simulink model "controller13_AIS"  (R2020b)
settings: Solver=FixedStepDiscrete  StartTime=0.0  StopTime=inf  RelTol=1e-3
values from neighbouring files (symbols this model uses):
  ctr = make_controller()    [setup_controller_with_functions.m]
  mdl = make_model(flight_time)    [setup_controller_with_functions.m]
  ukf_P0_flat = UKF.flatten_matrix(ukf_sys.P0)    [controller_setup_ukf.m]
  ukf_prediction_time = 0.015    [controller_setup_ukf.m]
  ukf_s0 = ukf_sys.s0    [controller_setup_ukf.m]
  ukf_sys = UKF.initialize_ukf_sys(rbt, mdl, ukf_params)    [controller_setup_ukf.m]
  ukf_use_prediction = 1    [controller_setup_ukf.m]
undefined symbols (not defined in the file or in its folder): ctr1, ctr2, DiscIntNeverNeededParam, flt, IO397, rbt1, rbt2, rsim1, rsim2, som, traj2
libraries: simulink x63, slrealtimeloglib x21, slrealtimetgmanagement x8, slrealtimeseriallib x5, speedgoatlib_fpga_analog_io x4, slrealtimeutilitieslib x3, dspfdesign x2, speedgoatlib_fpga x2, slrealtimeiplib x2, speedgoatlib_fpga_dio x1
(part 4 of 5)

== system controller13_AIS/Measurement manager 2/safety check system/landing condition ==
  z : Inport
  Add : Sum  Inputs=+--
  SaturatingRamp1 : DiscreteIntegrator  gainval=1  SampleTime=-1  UpperSaturationLimit=1  LowerSaturationLimit=0  ICPrevOutput=DiscIntNeverNeededParam  ICPrevScaledInput=DiscIntNeverNeededParam
  constant : Constant
  constant1 : Constant  Value=2
  constant2 : Constant  Value=mdl.i_delay
  landing_cond : MATLAB Function  TreatAsAtomicUnit=on  SystemSampleTime=mdl.T
  en : Outport
  wires:
  SaturatingRamp1/1 -> Add/1
  constant/1 -> SaturatingRamp1/1
  constant1/1 -> Add/2
  constant2/1 -> Add/3
  Add/1 -> landing_cond/2(time_cond)
  z/1 -> landing_cond/1(alt)
  landing_cond/1(en) -> en/1

== system controller13_AIS/signal generator 1/Bias_Signal/AveragedBias ==
  note: To avoid having signal "jump",
      | we want SMOOTH transitions
      | in frequency (i.e., a weighted sum
      | of current freq and freq some delta t ago)
  note: time constant = 0.002sec
  In1 : Inport
  Discrete Transfer Fcn : DiscreteTransferFcn  Numerator=[0.05]  Denominator=[1 -.95]
  Out1 : Outport
  wires:
  In1/1 -> Discrete Transfer Fcn/1
  Discrete Transfer Fcn/1 -> Out1/1

== system controller13_AIS/signal generator 1/Bias_Signal/SIgnalForRamp_binary ==
  note: Should output 1 or -1,
      | so signal ramps UP to 1
      | or DOWN to 0.
  In1 : Inport
  Add : Sum  Inputs=+-
  Compare To Zero : simulink/Logic and Bit Operations/Compare To Zero  relop=>  OutDataTypeStr=uint8  ZeroCross=off
  Constant : Constant
  Data Type Conversion : DataTypeConversion  OutDataTypeStr=double
  Gain : Gain  Gain=2
  Out1 : Outport
  wires:
  In1/1 -> Compare To Zero/1
  Compare To Zero/1 -> Data Type Conversion/1
  Gain/1 -> Add/1
  Constant/1 -> Add/2
  Add/1 -> Out1/1
  Data Type Conversion/1 -> Gain/1

== system controller13_AIS/signal generator 1/Drive_Signal1/AveragedAmp_filtered ==
  note: To avoid having signal "jump",
      | we want SMOOTH transitions
      | in frequency (i.e., a weighted sum
      | of current freq and freq some delta t ago)
  note: time constant 0.002sec
      | for 10kHz samping
  In1 : Inport
  Discrete Transfer Fcn : DiscreteTransferFcn  Numerator=[0.05]  Denominator=[1 -.95]
  Out1 : Outport
  wires:
  In1/1 -> Discrete Transfer Fcn/1
  Discrete Transfer Fcn/1 -> Out1/1

== system controller13_AIS/signal generator 1/Drive_Signal1/AveragedOffset_filtered ==
  note: To avoid having signal "jump",
      | we want SMOOTH transitions
      | in frequency (i.e., a weighted sum
      | of current freq and freq some delta t ago)
  note: c
  note: time constant 0.02sec
      | for 10kHz samping
  In1 : Inport
  Discrete Transfer Fcn : DiscreteTransferFcn  Numerator=[0.05]  Denominator=[1 -.95]
  Out1 : Outport
  wires:
  In1/1 -> Discrete Transfer Fcn/1
  Discrete Transfer Fcn/1 -> Out1/1

== system controller13_AIS/signal generator 1/Drive_Signal1/AveragedTau_filtered ==
  note: To avoid having signal "jump",
      | we want SMOOTH transitions
      | in frequency (i.e., a weighted sum
      | of current freq and freq some delta t ago)
  note: time constant 0.002sec
      | for 10kHz samping
  In1 : Inport
  Discrete Transfer Fcn : DiscreteTransferFcn  Numerator=[0.05]  Denominator=[1, -0.95]
  Out1 : Outport
  wires:
  In1/1 -> Discrete Transfer Fcn/1
  Discrete Transfer Fcn/1 -> Out1/1

== system controller13_AIS/signal generator 1/Drive_Signal1/SignalForRamp_binary ==
  note: Should output 1 or -1,
      | so signal ramps UP to 1
      | or DOWN to 0.
  In1 : Inport
  Add : Sum  Inputs=+-
  Compare To Zero : simulink/Logic and Bit Operations/Compare To Zero  relop=>  OutDataTypeStr=uint8  ZeroCross=off
  Constant : Constant
  Data Type Conversion : DataTypeConversion  OutDataTypeStr=double
  Gain : Gain  Gain=2
  Out1 : Outport
  wires:
  In1/1 -> Compare To Zero/1
  Compare To Zero/1 -> Data Type Conversion/1
  Gain/1 -> Add/1
  Constant/1 -> Add/2
  Add/1 -> Out1/1
  Data Type Conversion/1 -> Gain/1

== system controller13_AIS/signal generator 1/Drive_Signal1/SignalForSin_binary ==
  note: We want this to stay "high" for 1
      | second after the actual "enable"
      | is turned off...
  In1 : Inport
  Compare To Zero : simulink/Logic and Bit Operations/Compare To Zero  relop=>  OutDataTypeStr=uint8  ZeroCross=off
  Data Type Conversion : DataTypeConversion  OutDataTypeStr=double
  Out1 : Outport
  wires:
  In1/1 -> Compare To Zero/1
  Compare To Zero/1 -> Data Type Conversion/1
  Data Type Conversion/1 -> Out1/1

== system controller13_AIS/signal generator 1/Drive_Signal1/Subsystem ==
  note: positive value pushes the left wing forward
  split cycle mu : Inport
  In2 : Inport  Port=2
  1-mu : Sum  Inputs=+-
  2f : Gain  Gain=2
  2nd harmonic : Trigonometry  OutputSignalType=real
  2pi : Gain  Gain=2*pi
  Abs1 : Abs
  Add : Sum
  Constant : Constant
  combined sines : Sum
  deg to rad : Gain  Gain=pi/180
  f : Gain  Gain=-1
  first harmonic : Trigonometry  OutputSignalType=real
  omega*t : DiscreteIntegrator  SampleTime=-1  ICPrevOutput=DiscIntNeverNeededParam  ICPrevScaledInput=DiscIntNeverNeededParam
  phase offset : Constant  Value=0
  signal with gain1 : Product  RndMeth=Zero
  signal with gain2 : Product  RndMeth=Zero
  split cycle signal : Outport
  wires:
  2f/1 -> 2nd harmonic/1
  first harmonic/1 -> signal with gain1/2
  Constant/1 -> 1-mu/1
  split cycle mu/1 -> f/1, Abs1/1
  1-mu/1 -> signal with gain1/1
  2nd harmonic/1 -> signal with gain2/2
  signal with gain1/1 -> combined sines/1
  signal with gain2/1 -> combined sines/2
  combined sines/1 -> split cycle signal/1
  f/1 -> signal with gain2/1
  Abs1/1 -> 1-mu/2
  In2/1 -> 2pi/1
  2pi/1 -> omega*t/1
  omega*t/1 -> Add/2
  Add/1 -> first harmonic/1, 2f/1
  phase offset/1 -> deg to rad/1
  deg to rad/1 -> Add/1

== system controller13_AIS/signal generator 1/Drive_Signal2/AveragedAmp_filtered ==
  note: To avoid having signal "jump",
      | we want SMOOTH transitions
      | in frequency (i.e., a weighted sum
      | of current freq and freq some delta t ago)
  note: time constant 0.002sec
      | for 10kHz samping
  In1 : Inport
  Discrete Transfer Fcn : DiscreteTransferFcn  Numerator=[0.05]  Denominator=[1 -.95]
  Out1 : Outport
  wires:
  In1/1 -> Discrete Transfer Fcn/1
  Discrete Transfer Fcn/1 -> Out1/1

== system controller13_AIS/signal generator 1/Drive_Signal2/AveragedOffset_filtered ==
  note: To avoid having signal "jump",
      | we want SMOOTH transitions
      | in frequency (i.e., a weighted sum
      | of current freq and freq some delta t ago)
  note: c
  note: time constant 0.02sec
      | for 10kHz samping
  In1 : Inport
  Discrete Transfer Fcn : DiscreteTransferFcn  Numerator=[0.05]  Denominator=[1 -.95]
  Out1 : Outport
  wires:
  In1/1 -> Discrete Transfer Fcn/1
  Discrete Transfer Fcn/1 -> Out1/1

== system controller13_AIS/signal generator 1/Drive_Signal2/AveragedTau_filtered ==
  note: To avoid having signal "jump",
      | we want SMOOTH transitions
      | in frequency (i.e., a weighted sum
      | of current freq and freq some delta t ago)
  note: time constant 0.002sec
      | for 10kHz samping
  In1 : Inport
  Discrete Transfer Fcn : DiscreteTransferFcn  Numerator=[0.05]  Denominator=[1, -0.95]
  Out1 : Outport
  wires:
  In1/1 -> Discrete Transfer Fcn/1
  Discrete Transfer Fcn/1 -> Out1/1

== system controller13_AIS/signal generator 1/Drive_Signal2/SignalForRamp_binary ==
  note: Should output 1 or -1,
      | so signal ramps UP to 1
      | or DOWN to 0.
  In1 : Inport
  Add : Sum  Inputs=+-
  Compare To Zero : simulink/Logic and Bit Operations/Compare To Zero  relop=>  OutDataTypeStr=uint8  ZeroCross=off
  Constant : Constant
  Data Type Conversion : DataTypeConversion  OutDataTypeStr=double
  Gain : Gain  Gain=2
  Out1 : Outport
  wires:
  In1/1 -> Compare To Zero/1
  Compare To Zero/1 -> Data Type Conversion/1
  Gain/1 -> Add/1
  Constant/1 -> Add/2
  Add/1 -> Out1/1
  Data Type Conversion/1 -> Gain/1

== system controller13_AIS/signal generator 1/Drive_Signal2/SignalForSin_binary ==
  note: We want this to stay "high" for 1
      | second after the actual "enable"
      | is turned off...
  In1 : Inport
  Compare To Zero : simulink/Logic and Bit Operations/Compare To Zero  relop=>  OutDataTypeStr=uint8  ZeroCross=off
  Data Type Conversion : DataTypeConversion  OutDataTypeStr=double
  Out1 : Outport
  wires:
  In1/1 -> Compare To Zero/1
  Compare To Zero/1 -> Data Type Conversion/1
  Data Type Conversion/1 -> Out1/1

== system controller13_AIS/signal generator 1/Drive_Signal2/Subsystem ==
  note: positive value pushes the left wing forward
  split cycle mu : Inport
  In2 : Inport  Port=2
  1-mu : Sum  Inputs=+-
  2f : Gain  Gain=2
  2nd harmonic : Trigonometry  OutputSignalType=real
  2pi : Gain  Gain=2*pi
  Abs1 : Abs
  Add : Sum
  Constant : Constant
  combined sines : Sum
  deg to rad : Gain  Gain=pi/180
  f : Gain  Gain=-1
  first harmonic : Trigonometry  OutputSignalType=real
  omega*t : DiscreteIntegrator  SampleTime=-1  ICPrevOutput=DiscIntNeverNeededParam  ICPrevScaledInput=DiscIntNeverNeededParam
  phase offset : Constant  Value=0
  signal with gain1 : Product  RndMeth=Zero
  signal with gain2 : Product  RndMeth=Zero
  split cycle signal : Outport
  wires:
  2f/1 -> 2nd harmonic/1
  first harmonic/1 -> signal with gain1/2
  Constant/1 -> 1-mu/1
  split cycle mu/1 -> f/1, Abs1/1
  1-mu/1 -> signal with gain1/1
  2nd harmonic/1 -> signal with gain2/2
  signal with gain1/1 -> combined sines/1
  signal with gain2/1 -> combined sines/2
  combined sines/1 -> split cycle signal/1
  f/1 -> signal with gain2/1
  Abs1/1 -> 1-mu/2
  In2/1 -> 2pi/1
  2pi/1 -> omega*t/1
  omega*t/1 -> Add/2
  Add/1 -> first harmonic/1, 2f/1
  phase offset/1 -> deg to rad/1
  deg to rad/1 -> Add/1

== system controller13_AIS/signal generator 1/Drive_Signal3/AveragedAmp_filtered ==
  note: To avoid having signal "jump",
      | we want SMOOTH transitions
      | in frequency (i.e., a weighted sum
      | of current freq and freq some delta t ago)
  note: time constant 0.002sec
      | for 10kHz samping
  In1 : Inport
  Discrete Transfer Fcn : DiscreteTransferFcn  Numerator=[0.05]  Denominator=[1 -.95]
  Out1 : Outport
  wires:
  In1/1 -> Discrete Transfer Fcn/1
  Discrete Transfer Fcn/1 -> Out1/1

== system controller13_AIS/signal generator 1/Drive_Signal3/AveragedOffset_filtered ==
  note: To avoid having signal "jump",
      | we want SMOOTH transitions
      | in frequency (i.e., a weighted sum
      | of current freq and freq some delta t ago)
  note: c
  note: time constant 0.02sec
      | for 10kHz samping
  In1 : Inport
  Discrete Transfer Fcn : DiscreteTransferFcn  Numerator=[0.05]  Denominator=[1 -.95]
  Out1 : Outport
  wires:
  In1/1 -> Discrete Transfer Fcn/1
  Discrete Transfer Fcn/1 -> Out1/1

== system controller13_AIS/signal generator 1/Drive_Signal3/AveragedTau_filtered ==
  note: To avoid having signal "jump",
      | we want SMOOTH transitions
      | in frequency (i.e., a weighted sum
      | of current freq and freq some delta t ago)
  note: time constant 0.002sec
      | for 10kHz samping
  In1 : Inport
  Discrete Transfer Fcn : DiscreteTransferFcn  Numerator=[0.05]  Denominator=[1 -.95]
  Out1 : Outport
  wires:
  In1/1 -> Discrete Transfer Fcn/1
  Discrete Transfer Fcn/1 -> Out1/1

== system controller13_AIS/signal generator 1/Drive_Signal3/SignalForRamp_binary ==
  note: Should output 1 or -1,
      | so signal ramps UP to 1
      | or DOWN to 0.
  In1 : Inport
  Add : Sum  Inputs=+-
  Compare To Zero : simulink/Logic and Bit Operations/Compare To Zero  relop=>  OutDataTypeStr=uint8  ZeroCross=off
  Constant : Constant
  Data Type Conversion : DataTypeConversion  OutDataTypeStr=double
  Gain : Gain  Gain=2
  Out1 : Outport
  wires:
  In1/1 -> Compare To Zero/1
  Compare To Zero/1 -> Data Type Conversion/1
  Gain/1 -> Add/1
  Constant/1 -> Add/2
  Add/1 -> Out1/1
  Data Type Conversion/1 -> Gain/1

== system controller13_AIS/signal generator 1/Drive_Signal3/SignalForSin_binary ==
  note: We want this to stay "high" for 1
      | second after the actual "enable"
      | is turned off...
  In1 : Inport
  Compare To Zero : simulink/Logic and Bit Operations/Compare To Zero  relop=>  OutDataTypeStr=uint8  ZeroCross=off
  Data Type Conversion : DataTypeConversion  OutDataTypeStr=double
  Out1 : Outport
  wires:
  In1/1 -> Compare To Zero/1
  Compare To Zero/1 -> Data Type Conversion/1
  Data Type Conversion/1 -> Out1/1

== system controller13_AIS/signal generator 1/Drive_Signal3/Subsystem ==
  split cycle mu : Inport
  In2 : Inport  Port=2
  1-mu : Sum  Inputs=+-
  2f : Gain  Gain=2
  2nd harmonic : Trigonometry  OutputSignalType=real
  2pi : Gain  Gain=2*pi
  Abs1 : Abs
  Constant : Constant
  SmoothClock : DiscreteIntegrator  SampleTime=-1  ICPrevOutput=DiscIntNeverNeededParam  ICPrevScaledInput=DiscIntNeverNeededParam
  combined sines : Sum
  f : Gain
  first harmonic : Trigonometry  OutputSignalType=real
  signal with gain1 : Product  RndMeth=Zero
  signal with gain2 : Product  RndMeth=Zero
  split cycle signal : Outport
  wires:
  SmoothClock/1 -> first harmonic/1, 2f/1
  2f/1 -> 2nd harmonic/1
  2pi/1 -> SmoothClock/1
  first harmonic/1 -> signal with gain1/2
  Constant/1 -> 1-mu/1
  split cycle mu/1 -> f/1, Abs1/1
  1-mu/1 -> signal with gain1/1
  2nd harmonic/1 -> signal with gain2/2
  signal with gain1/1 -> combined sines/1
  signal with gain2/1 -> combined sines/2
  combined sines/1 -> split cycle signal/1
  In2/1 -> 2pi/1
  f/1 -> signal with gain2/1
  Abs1/1 -> 1-mu/2

== system controller13_AIS/signal generator 1/Drive_Signal4/AveragedAmp_filtered ==
  note: To avoid having signal "jump",
      | we want SMOOTH transitions
      | in frequency (i.e., a weighted sum
      | of current freq and freq some delta t ago)
  note: time constant 0.002sec
      | for 10kHz samping
  In1 : Inport
  Discrete Transfer Fcn : DiscreteTransferFcn  Numerator=[0.05]  Denominator=[1 -.95]
  Out1 : Outport
  wires:
  In1/1 -> Discrete Transfer Fcn/1
  Discrete Transfer Fcn/1 -> Out1/1

== system controller13_AIS/signal generator 1/Drive_Signal4/AveragedOffset_filtered ==
  note: To avoid having signal "jump",
      | we want SMOOTH transitions
      | in frequency (i.e., a weighted sum
      | of current freq and freq some delta t ago)
  note: c
  note: time constant 0.02sec
      | for 10kHz samping
  In1 : Inport
  Discrete Transfer Fcn : DiscreteTransferFcn  Numerator=[0.05]  Denominator=[1 -.95]
  Out1 : Outport
  wires:
  In1/1 -> Discrete Transfer Fcn/1
  Discrete Transfer Fcn/1 -> Out1/1

== system controller13_AIS/signal generator 1/Drive_Signal4/AveragedTau_filtered ==
  note: To avoid having signal "jump",
      | we want SMOOTH transitions
      | in frequency (i.e., a weighted sum
      | of current freq and freq some delta t ago)
  note: time constant 0.002sec
      | for 10kHz samping
  In1 : Inport
  Discrete Transfer Fcn : DiscreteTransferFcn  Numerator=[0.05]  Denominator=[1, -0.95]
  Out1 : Outport
  wires:
  In1/1 -> Discrete Transfer Fcn/1
  Discrete Transfer Fcn/1 -> Out1/1

== system controller13_AIS/signal generator 1/Drive_Signal4/SignalForRamp_binary ==
  note: Should output 1 or -1,
      | so signal ramps UP to 1
      | or DOWN to 0.
  In1 : Inport
  Add : Sum  Inputs=+-
  Compare To Zero : simulink/Logic and Bit Operations/Compare To Zero  relop=>  OutDataTypeStr=uint8  ZeroCross=off
  Constant : Constant
  Data Type Conversion : DataTypeConversion  OutDataTypeStr=double
  Gain : Gain  Gain=2
  Out1 : Outport
  wires:
  In1/1 -> Compare To Zero/1
  Compare To Zero/1 -> Data Type Conversion/1
  Gain/1 -> Add/1
  Constant/1 -> Add/2
  Add/1 -> Out1/1
  Data Type Conversion/1 -> Gain/1

== system controller13_AIS/signal generator 1/Drive_Signal4/SignalForSin_binary ==
  note: We want this to stay "high" for 1
      | second after the actual "enable"
      | is turned off...
  In1 : Inport
  Compare To Zero : simulink/Logic and Bit Operations/Compare To Zero  relop=>  OutDataTypeStr=uint8  ZeroCross=off
  Data Type Conversion : DataTypeConversion  OutDataTypeStr=double
  Out1 : Outport
  wires:
  In1/1 -> Compare To Zero/1
  Compare To Zero/1 -> Data Type Conversion/1
  Data Type Conversion/1 -> Out1/1

== system controller13_AIS/signal generator 1/Drive_Signal4/Subsystem ==
  note: positive value pushes the left wing forward
  split cycle mu : Inport
  In2 : Inport  Port=2
  1-mu : Sum  Inputs=+-
  2f : Gain  Gain=2
  2nd harmonic : Trigonometry  OutputSignalType=real
  2pi : Gain  Gain=2*pi
  Abs1 : Abs
  Add : Sum
  Constant : Constant
  combined sines : Sum
  deg to rad : Gain  Gain=pi/180
  f : Gain  Gain=-1
  first harmonic : Trigonometry  OutputSignalType=real
  omega*t : DiscreteIntegrator  SampleTime=-1  ICPrevOutput=DiscIntNeverNeededParam  ICPrevScaledInput=DiscIntNeverNeededParam
  phase offset : Constant  Value=0
  signal with gain1 : Product  RndMeth=Zero
  signal with gain2 : Product  RndMeth=Zero
  split cycle signal : Outport
  wires:
  2f/1 -> 2nd harmonic/1
  first harmonic/1 -> signal with gain1/2
  Constant/1 -> 1-mu/1
  split cycle mu/1 -> f/1, Abs1/1
  1-mu/1 -> signal with gain1/1
  2nd harmonic/1 -> signal with gain2/2
  signal with gain1/1 -> combined sines/1
  signal with gain2/1 -> combined sines/2
  combined sines/1 -> split cycle signal/1
  f/1 -> signal with gain2/1
  Abs1/1 -> 1-mu/2
  In2/1 -> 2pi/1
  2pi/1 -> omega*t/1
  omega*t/1 -> Add/2
  Add/1 -> first harmonic/1, 2f/1
  phase offset/1 -> deg to rad/1
  deg to rad/1 -> Add/1

== system controller13_AIS/signal generator1/Bias_Signal/AveragedBias ==
  note: To avoid having signal "jump",
      | we want SMOOTH transitions
      | in frequency (i.e., a weighted sum
      | of current freq and freq some delta t ago)
  note: time constant = 0.002sec
  In1 : Inport
  Discrete Transfer Fcn : DiscreteTransferFcn  Numerator=[0.05]  Denominator=[1 -.95]
  Out1 : Outport
  wires:
  In1/1 -> Discrete Transfer Fcn/1
  Discrete Transfer Fcn/1 -> Out1/1

== system controller13_AIS/signal generator1/Bias_Signal/SIgnalForRamp_binary ==
  note: Should output 1 or -1,
      | so signal ramps UP to 1
      | or DOWN to 0.
  In1 : Inport
  Add : Sum  Inputs=+-
  Compare To Zero : simulink/Logic and Bit Operations/Compare To Zero  relop=>  OutDataTypeStr=uint8  ZeroCross=off
  Constant : Constant
  Data Type Conversion : DataTypeConversion  OutDataTypeStr=double
  Gain : Gain  Gain=2
  Out1 : Outport
  wires:
  In1/1 -> Compare To Zero/1
  Compare To Zero/1 -> Data Type Conversion/1
  Gain/1 -> Add/1
  Constant/1 -> Add/2
  Add/1 -> Out1/1
  Data Type Conversion/1 -> Gain/1

== system controller13_AIS/signal generator1/Drive_Signal1/AveragedAmp_filtered ==
  note: To avoid having signal "jump",
      | we want SMOOTH transitions
      | in frequency (i.e., a weighted sum
      | of current freq and freq some delta t ago)
  note: time constant 0.002sec
      | for 10kHz samping
  In1 : Inport
  Discrete Transfer Fcn : DiscreteTransferFcn  Numerator=[0.05]  Denominator=[1 -.95]
  Out1 : Outport
  wires:
  In1/1 -> Discrete Transfer Fcn/1
  Discrete Transfer Fcn/1 -> Out1/1

== system controller13_AIS/signal generator1/Drive_Signal1/AveragedOffset_filtered ==
  note: To avoid having signal "jump",
      | we want SMOOTH transitions
      | in frequency (i.e., a weighted sum
      | of current freq and freq some delta t ago)
  note: c
  note: time constant 0.02sec
      | for 10kHz samping
  In1 : Inport
  Discrete Transfer Fcn : DiscreteTransferFcn  Numerator=[0.05]  Denominator=[1 -.95]
  Out1 : Outport
  wires:
  In1/1 -> Discrete Transfer Fcn/1
  Discrete Transfer Fcn/1 -> Out1/1

== system controller13_AIS/signal generator1/Drive_Signal1/AveragedTau_filtered ==
  note: To avoid having signal "jump",
      | we want SMOOTH transitions
      | in frequency (i.e., a weighted sum
      | of current freq and freq some delta t ago)
  note: time constant 0.002sec
      | for 10kHz samping
  In1 : Inport
  Discrete Transfer Fcn : DiscreteTransferFcn  Numerator=[0.05]  Denominator=[1, -0.95]
  Out1 : Outport
  wires:
  In1/1 -> Discrete Transfer Fcn/1
  Discrete Transfer Fcn/1 -> Out1/1

== system controller13_AIS/signal generator1/Drive_Signal1/SignalForRamp_binary ==
  note: Should output 1 or -1,
      | so signal ramps UP to 1
      | or DOWN to 0.
  In1 : Inport
  Add : Sum  Inputs=+-
  Compare To Zero : simulink/Logic and Bit Operations/Compare To Zero  relop=>  OutDataTypeStr=uint8  ZeroCross=off
  Constant : Constant
  Data Type Conversion : DataTypeConversion  OutDataTypeStr=double
  Gain : Gain  Gain=2
  Out1 : Outport
  wires:
  In1/1 -> Compare To Zero/1
  Compare To Zero/1 -> Data Type Conversion/1
  Gain/1 -> Add/1
  Constant/1 -> Add/2
  Add/1 -> Out1/1
  Data Type Conversion/1 -> Gain/1

== system controller13_AIS/signal generator1/Drive_Signal1/SignalForSin_binary ==
  note: We want this to stay "high" for 1
      | second after the actual "enable"
      | is turned off...
  In1 : Inport
  Compare To Zero : simulink/Logic and Bit Operations/Compare To Zero  relop=>  OutDataTypeStr=uint8  ZeroCross=off
  Data Type Conversion : DataTypeConversion  OutDataTypeStr=double
  Out1 : Outport
  wires:
  In1/1 -> Compare To Zero/1
  Compare To Zero/1 -> Data Type Conversion/1
  Data Type Conversion/1 -> Out1/1

== system controller13_AIS/signal generator1/Drive_Signal1/Subsystem ==
  note: positive value pushes the left wing forward
  split cycle mu : Inport
  In2 : Inport  Port=2
  1-mu : Sum  Inputs=+-
  2f : Gain  Gain=2
  2nd harmonic : Trigonometry  OutputSignalType=real
  2pi : Gain  Gain=2*pi
  Abs1 : Abs
  Add : Sum
  Constant : Constant
  combined sines : Sum
  deg to rad : Gain  Gain=pi/180
  f : Gain  Gain=-1
  first harmonic : Trigonometry  OutputSignalType=real
  omega*t : DiscreteIntegrator  SampleTime=-1  ICPrevOutput=DiscIntNeverNeededParam  ICPrevScaledInput=DiscIntNeverNeededParam
  phase offset : Constant  Value=0
  signal with gain1 : Product  RndMeth=Zero
  signal with gain2 : Product  RndMeth=Zero
  split cycle signal : Outport
  wires:
  2f/1 -> 2nd harmonic/1
  first harmonic/1 -> signal with gain1/2
  Constant/1 -> 1-mu/1
  split cycle mu/1 -> f/1, Abs1/1
  1-mu/1 -> signal with gain1/1
  2nd harmonic/1 -> signal with gain2/2
  signal with gain1/1 -> combined sines/1
  signal with gain2/1 -> combined sines/2
  combined sines/1 -> split cycle signal/1
  f/1 -> signal with gain2/1
  Abs1/1 -> 1-mu/2
  In2/1 -> 2pi/1
  2pi/1 -> omega*t/1
  omega*t/1 -> Add/2
  Add/1 -> first harmonic/1, 2f/1
  phase offset/1 -> deg to rad/1
  deg to rad/1 -> Add/1

== system controller13_AIS/signal generator1/Drive_Signal2/AveragedAmp_filtered ==
  note: To avoid having signal "jump",
      | we want SMOOTH transitions
      | in frequency (i.e., a weighted sum
      | of current freq and freq some delta t ago)
  note: time constant 0.002sec
      | for 10kHz samping
  In1 : Inport
  Discrete Transfer Fcn : DiscreteTransferFcn  Numerator=[0.05]  Denominator=[1 -.95]
  Out1 : Outport
  wires:
  In1/1 -> Discrete Transfer Fcn/1
  Discrete Transfer Fcn/1 -> Out1/1

== system controller13_AIS/signal generator1/Drive_Signal2/AveragedOffset_filtered ==
  note: To avoid having signal "jump",
      | we want SMOOTH transitions
      | in frequency (i.e., a weighted sum
      | of current freq and freq some delta t ago)
  note: c
  note: time constant 0.02sec
      | for 10kHz samping
  In1 : Inport
  Discrete Transfer Fcn : DiscreteTransferFcn  Numerator=[0.05]  Denominator=[1 -.95]
  Out1 : Outport
  wires:
  In1/1 -> Discrete Transfer Fcn/1
  Discrete Transfer Fcn/1 -> Out1/1

== system controller13_AIS/signal generator1/Drive_Signal2/AveragedTau_filtered ==
  note: To avoid having signal "jump",
      | we want SMOOTH transitions
      | in frequency (i.e., a weighted sum
      | of current freq and freq some delta t ago)
  note: time constant 0.002sec
      | for 10kHz samping
  In1 : Inport
  Discrete Transfer Fcn : DiscreteTransferFcn  Numerator=[0.05]  Denominator=[1, -0.95]
  Out1 : Outport
  wires:
  In1/1 -> Discrete Transfer Fcn/1
  Discrete Transfer Fcn/1 -> Out1/1

== system controller13_AIS/signal generator1/Drive_Signal2/SignalForRamp_binary ==
  note: Should output 1 or -1,
      | so signal ramps UP to 1
      | or DOWN to 0.
  In1 : Inport
  Add : Sum  Inputs=+-
  Compare To Zero : simulink/Logic and Bit Operations/Compare To Zero  relop=>  OutDataTypeStr=uint8  ZeroCross=off
  Constant : Constant
  Data Type Conversion : DataTypeConversion  OutDataTypeStr=double
  Gain : Gain  Gain=2
  Out1 : Outport
  wires:
  In1/1 -> Compare To Zero/1
  Compare To Zero/1 -> Data Type Conversion/1
  Gain/1 -> Add/1
  Constant/1 -> Add/2
  Add/1 -> Out1/1
  Data Type Conversion/1 -> Gain/1

== system controller13_AIS/signal generator1/Drive_Signal2/SignalForSin_binary ==
  note: We want this to stay "high" for 1
      | second after the actual "enable"
      | is turned off...
  In1 : Inport
  Compare To Zero : simulink/Logic and Bit Operations/Compare To Zero  relop=>  OutDataTypeStr=uint8  ZeroCross=off
  Data Type Conversion : DataTypeConversion  OutDataTypeStr=double
  Out1 : Outport
  wires:
  In1/1 -> Compare To Zero/1
  Compare To Zero/1 -> Data Type Conversion/1
  Data Type Conversion/1 -> Out1/1

== system controller13_AIS/signal generator1/Drive_Signal2/Subsystem ==
  note: positive value pushes the left wing forward
  split cycle mu : Inport
  In2 : Inport  Port=2
  1-mu : Sum  Inputs=+-
  2f : Gain  Gain=2
  2nd harmonic : Trigonometry  OutputSignalType=real
  2pi : Gain  Gain=2*pi
  Abs1 : Abs
  Add : Sum
  Constant : Constant
  combined sines : Sum
  deg to rad : Gain  Gain=pi/180
  f : Gain  Gain=-1
  first harmonic : Trigonometry  OutputSignalType=real
  omega*t : DiscreteIntegrator  SampleTime=-1  ICPrevOutput=DiscIntNeverNeededParam  ICPrevScaledInput=DiscIntNeverNeededParam
  phase offset : Constant  Value=0
  signal with gain1 : Product  RndMeth=Zero
  signal with gain2 : Product  RndMeth=Zero
  split cycle signal : Outport
  wires:
  2f/1 -> 2nd harmonic/1
  first harmonic/1 -> signal with gain1/2
  Constant/1 -> 1-mu/1
  split cycle mu/1 -> f/1, Abs1/1
  1-mu/1 -> signal with gain1/1
  2nd harmonic/1 -> signal with gain2/2
  signal with gain1/1 -> combined sines/1
  signal with gain2/1 -> combined sines/2
  combined sines/1 -> split cycle signal/1
  f/1 -> signal with gain2/1
  Abs1/1 -> 1-mu/2
  In2/1 -> 2pi/1
  2pi/1 -> omega*t/1
  omega*t/1 -> Add/2
  Add/1 -> first harmonic/1, 2f/1
  phase offset/1 -> deg to rad/1
  deg to rad/1 -> Add/1

== system controller13_AIS/signal generator1/Drive_Signal3/AveragedAmp_filtered ==
  note: To avoid having signal "jump",
      | we want SMOOTH transitions
      | in frequency (i.e., a weighted sum
      | of current freq and freq some delta t ago)
  note: time constant 0.002sec
      | for 10kHz samping
  In1 : Inport
  Discrete Transfer Fcn : DiscreteTransferFcn  Numerator=[0.05]  Denominator=[1 -.95]
  Out1 : Outport
  wires:
  In1/1 -> Discrete Transfer Fcn/1
  Discrete Transfer Fcn/1 -> Out1/1

== system controller13_AIS/signal generator1/Drive_Signal3/AveragedOffset_filtered ==
  note: To avoid having signal "jump",
      | we want SMOOTH transitions
      | in frequency (i.e., a weighted sum
      | of current freq and freq some delta t ago)
  note: c
  note: time constant 0.02sec
      | for 10kHz samping
  In1 : Inport
  Discrete Transfer Fcn : DiscreteTransferFcn  Numerator=[0.05]  Denominator=[1 -.95]
  Out1 : Outport
  wires:
  In1/1 -> Discrete Transfer Fcn/1
  Discrete Transfer Fcn/1 -> Out1/1

== system controller13_AIS/signal generator1/Drive_Signal3/AveragedTau_filtered ==
  note: To avoid having signal "jump",
      | we want SMOOTH transitions
      | in frequency (i.e., a weighted sum
      | of current freq and freq some delta t ago)
  note: time constant 0.002sec
      | for 10kHz samping
  In1 : Inport
  Discrete Transfer Fcn : DiscreteTransferFcn  Numerator=[0.05]  Denominator=[1 -.95]
  Out1 : Outport
  wires:
  In1/1 -> Discrete Transfer Fcn/1
  Discrete Transfer Fcn/1 -> Out1/1

== system controller13_AIS/signal generator1/Drive_Signal3/SignalForRamp_binary ==
  note: Should output 1 or -1,
      | so signal ramps UP to 1
      | or DOWN to 0.
  In1 : Inport
  Add : Sum  Inputs=+-
  Compare To Zero : simulink/Logic and Bit Operations/Compare To Zero  relop=>  OutDataTypeStr=uint8  ZeroCross=off
  Constant : Constant
  Data Type Conversion : DataTypeConversion  OutDataTypeStr=double
  Gain : Gain  Gain=2
  Out1 : Outport
  wires:
  In1/1 -> Compare To Zero/1
  Compare To Zero/1 -> Data Type Conversion/1
  Gain/1 -> Add/1
  Constant/1 -> Add/2
  Add/1 -> Out1/1
  Data Type Conversion/1 -> Gain/1

== system controller13_AIS/signal generator1/Drive_Signal3/SignalForSin_binary ==
  note: We want this to stay "high" for 1
      | second after the actual "enable"
      | is turned off...
  In1 : Inport
  Compare To Zero : simulink/Logic and Bit Operations/Compare To Zero  relop=>  OutDataTypeStr=uint8  ZeroCross=off
  Data Type Conversion : DataTypeConversion  OutDataTypeStr=double
  Out1 : Outport
  wires:
  In1/1 -> Compare To Zero/1
  Compare To Zero/1 -> Data Type Conversion/1
  Data Type Conversion/1 -> Out1/1

== system controller13_AIS/signal generator1/Drive_Signal3/Subsystem ==
  split cycle mu : Inport
  In2 : Inport  Port=2
  1-mu : Sum  Inputs=+-
  2f : Gain  Gain=2
  2nd harmonic : Trigonometry  OutputSignalType=real
  2pi : Gain  Gain=2*pi
  Abs1 : Abs
  Constant : Constant
  SmoothClock : DiscreteIntegrator  SampleTime=-1  ICPrevOutput=DiscIntNeverNeededParam  ICPrevScaledInput=DiscIntNeverNeededParam
  combined sines : Sum
  f : Gain
  first harmonic : Trigonometry  OutputSignalType=real
  signal with gain1 : Product  RndMeth=Zero
  signal with gain2 : Product  RndMeth=Zero
  split cycle signal : Outport
  wires:
  SmoothClock/1 -> first harmonic/1, 2f/1
  2f/1 -> 2nd harmonic/1
  2pi/1 -> SmoothClock/1
  first harmonic/1 -> signal with gain1/2
  Constant/1 -> 1-mu/1
  split cycle mu/1 -> f/1, Abs1/1
  1-mu/1 -> signal with gain1/1
  2nd harmonic/1 -> signal with gain2/2
  signal with gain1/1 -> combined sines/1
  signal with gain2/1 -> combined sines/2
  combined sines/1 -> split cycle signal/1
  In2/1 -> 2pi/1
  f/1 -> signal with gain2/1
  Abs1/1 -> 1-mu/2

== system controller13_AIS/signal generator1/Drive_Signal4/AveragedAmp_filtered ==
  note: To avoid having signal "jump",
      | we want SMOOTH transitions
      | in frequency (i.e., a weighted sum
      | of current freq and freq some delta t ago)
  note: time constant 0.002sec
      | for 10kHz samping
  In1 : Inport
  Discrete Transfer Fcn : DiscreteTransferFcn  Numerator=[0.05]  Denominator=[1 -.95]
  Out1 : Outport
  wires:
  In1/1 -> Discrete Transfer Fcn/1
  Discrete Transfer Fcn/1 -> Out1/1

== system controller13_AIS/signal generator1/Drive_Signal4/AveragedOffset_filtered ==
  note: To avoid having signal "jump",
      | we want SMOOTH transitions
      | in frequency (i.e., a weighted sum
      | of current freq and freq some delta t ago)
  note: c
  note: time constant 0.02sec
      | for 10kHz samping
  In1 : Inport
  Discrete Transfer Fcn : DiscreteTransferFcn  Numerator=[0.05]  Denominator=[1 -.95]
  Out1 : Outport
  wires:
  In1/1 -> Discrete Transfer Fcn/1
  Discrete Transfer Fcn/1 -> Out1/1

== system controller13_AIS/signal generator1/Drive_Signal4/AveragedTau_filtered ==
  note: To avoid having signal "jump",
      | we want SMOOTH transitions
      | in frequency (i.e., a weighted sum
      | of current freq and freq some delta t ago)
  note: time constant 0.002sec
      | for 10kHz samping
  In1 : Inport
  Discrete Transfer Fcn : DiscreteTransferFcn  Numerator=[0.05]  Denominator=[1, -0.95]
  Out1 : Outport
  wires:
  In1/1 -> Discrete Transfer Fcn/1
  Discrete Transfer Fcn/1 -> Out1/1

== system controller13_AIS/signal generator1/Drive_Signal4/SignalForRamp_binary ==
  note: Should output 1 or -1,
      | so signal ramps UP to 1
      | or DOWN to 0.
  In1 : Inport
  Add : Sum  Inputs=+-
  Compare To Zero : simulink/Logic and Bit Operations/Compare To Zero  relop=>  OutDataTypeStr=uint8  ZeroCross=off
  Constant : Constant
  Data Type Conversion : DataTypeConversion  OutDataTypeStr=double
  Gain : Gain  Gain=2
  Out1 : Outport
  wires:
  In1/1 -> Compare To Zero/1
  Compare To Zero/1 -> Data Type Conversion/1
  Gain/1 -> Add/1
  Constant/1 -> Add/2
  Add/1 -> Out1/1
  Data Type Conversion/1 -> Gain/1

== system controller13_AIS/signal generator1/Drive_Signal4/SignalForSin_binary ==
  note: We want this to stay "high" for 1
      | second after the actual "enable"
      | is turned off...
  In1 : Inport
  Compare To Zero : simulink/Logic and Bit Operations/Compare To Zero  relop=>  OutDataTypeStr=uint8  ZeroCross=off
  Data Type Conversion : DataTypeConversion  OutDataTypeStr=double
  Out1 : Outport
  wires:
  In1/1 -> Compare To Zero/1
  Compare To Zero/1 -> Data Type Conversion/1
  Data Type Conversion/1 -> Out1/1

== system controller13_AIS/signal generator1/Drive_Signal4/Subsystem ==
  note: positive value pushes the left wing forward
  split cycle mu : Inport
  In2 : Inport  Port=2
  1-mu : Sum  Inputs=+-
  2f : Gain  Gain=2
  2nd harmonic : Trigonometry  OutputSignalType=real
  2pi : Gain  Gain=2*pi
  Abs1 : Abs
  Add : Sum
  Constant : Constant
  combined sines : Sum
  deg to rad : Gain  Gain=pi/180
  f : Gain  Gain=-1
  first harmonic : Trigonometry  OutputSignalType=real
  omega*t : DiscreteIntegrator  SampleTime=-1  ICPrevOutput=DiscIntNeverNeededParam  ICPrevScaledInput=DiscIntNeverNeededParam
  phase offset : Constant  Value=0
  signal with gain1 : Product  RndMeth=Zero
  signal with gain2 : Product  RndMeth=Zero
  split cycle signal : Outport
  wires:
  2f/1 -> 2nd harmonic/1
  first harmonic/1 -> signal with gain1/2
  Constant/1 -> 1-mu/1
  split cycle mu/1 -> f/1, Abs1/1
  1-mu/1 -> signal with gain1/1
  2nd harmonic/1 -> signal with gain2/2
  signal with gain1/1 -> combined sines/1
  signal with gain2/1 -> combined sines/2
  combined sines/1 -> split cycle signal/1
  f/1 -> signal with gain2/1
  Abs1/1 -> 1-mu/2
  In2/1 -> 2pi/1
  2pi/1 -> omega*t/1
  omega*t/1 -> Add/2
  Add/1 -> first harmonic/1, 2f/1
  phase offset/1 -> deg to rad/1
  deg to rad/1 -> Add/1

== system controller13_AIS/Adaptive Controller 1/adaptive system/integrator/safety2 ==
  In1 : Inport
  Compare To Constant1 : simulink/Logic and Bit Operations/Compare To Constant  relop=<=  const=inf  OutDataTypeStr=uint8
  Switch1 : Switch  Threshold=0.5
  zero1 : Constant  Value=0
  Out1 : Outport
  wires:
  In1/1 -> Switch1/1, Compare To Constant1/1
  Compare To Constant1/1 -> Switch1/2
  zero1/1 -> Switch1/3
  Switch1/1 -> Out1/1

== system controller13_AIS/Adaptive Controller 1/adaptive system/integrator/start ramp ==
  0.8 : Constant  Value=mdl.s_delay
  2 : Constant  Value=mdl.i_delay
  Add1 : Sum
  Add2 : Sum  Inputs=+-
  Compare To Zero : simulink/Logic and Bit Operations/Compare To Zero  relop=>  OutDataTypeStr=uint8  ZeroCross=off
  Data Type Conversion : DataTypeConversion
  constant : Constant
  counter : DiscreteIntegrator  gainval=1  SampleTime=-1  UpperSaturationLimit=1  LowerSaturationLimit=0  ICPrevOutput=DiscIntNeverNeededParam  ICPrevScaledInput=DiscIntNeverNeededParam
  saturation ramp : DiscreteIntegrator  gainval=5  SampleTime=-1  LimitOutput=on  UpperSaturationLimit=1  LowerSaturationLimit=-1  ICPrevOutput=DiscIntNeverNeededParam  ICPrevScaledInput=DiscIntNeverNeededParam
  Out1 : Outport
  wires:
  constant/1 -> counter/1
  2/1 -> Add1/1
  0.8/1 -> Add1/2
  counter/1 -> Add2/1
  Add1/1 -> Add2/2
  Add2/1 -> Compare To Zero/1
  Compare To Zero/1 -> Data Type Conversion/1
  saturation ramp/1 -> Out1/1
  Data Type Conversion/1 -> saturation ramp/1

== system controller13_AIS/Adaptive Controller 1/attitude and thrust controller/Yaw Controller/start ramp ==
  0.8 : Constant  Value=0.01
  2 : Constant  Value=mdl.i_delay
  Add1 : Sum
  Add2 : Sum  Inputs=+-
  Compare To Zero : simulink/Logic and Bit Operations/Compare To Zero  relop=>  OutDataTypeStr=uint8  ZeroCross=off
  Data Type Conversion : DataTypeConversion
  constant : Constant
  counter : DiscreteIntegrator  gainval=1  SampleTime=-1  UpperSaturationLimit=1  LowerSaturationLimit=0  ICPrevOutput=DiscIntNeverNeededParam  ICPrevScaledInput=DiscIntNeverNeededParam
  saturation ramp : DiscreteIntegrator  gainval=5  SampleTime=-1  LimitOutput=on  UpperSaturationLimit=1  LowerSaturationLimit=-1  ICPrevOutput=DiscIntNeverNeededParam  ICPrevScaledInput=DiscIntNeverNeededParam
  Out1 : Outport
  wires:
  constant/1 -> counter/1
  2/1 -> Add1/1
  0.8/1 -> Add1/2
  counter/1 -> Add2/1
  Add1/1 -> Add2/2
  Add2/1 -> Compare To Zero/1
  Compare To Zero/1 -> Data Type Conversion/1
  saturation ramp/1 -> Out1/1
  Data Type Conversion/1 -> saturation ramp/1

== system controller13_AIS/Adaptive Controller 1/observer/Rotaion/filtered derivative ==
  In1 : Inport
  att_s : Gain  Gain=mdl.f1
  filtered derivative : simulink/Discrete/Transfer Fcn Lead or Lag  PoleZ=mdl.zf1  ZeroZ=1  ICPrevOutput=0.0  ICPrevInput=0.0  DoSatur=off
      settings: SourceProductBaseCode=SL
  low pass3 : DiscreteTransferFcn  Numerator=mdl.vlp.n  Denominator=mdl.vlp.d
  Out1 : Outport
  wires:
  filtered derivative/1 -> low pass3/1
  att_s/1 -> filtered derivative/1
  In1/1 -> att_s/1
  low pass3/1 -> Out1/1

== system controller13_AIS/Adaptive Controller 1/observer/lateral observer/saturation ==
  In1 : Inport
  MinMax2 : MinMax  Inputs=2
  MinMax3 : MinMax  Function=max  Inputs=2
  lw1 : Constant  Value=-mdl.fd_lim
  up1 : Constant  Value=mdl.fd_lim
  Out1 : Outport
  wires:
  In1/1 -> MinMax2/2
  up1/1 -> MinMax2/1
  lw1/1 -> MinMax3/1
  MinMax2/1 -> MinMax3/2
  MinMax3/1 -> Out1/1

== system controller13_AIS/Adaptive Controller 2/adaptive system/integrator/safety2 ==
  In1 : Inport
  Compare To Constant1 : simulink/Logic and Bit Operations/Compare To Constant  relop=<=  const=inf  OutDataTypeStr=uint8
  Switch1 : Switch  Threshold=0.5
  zero1 : Constant  Value=0
  Out1 : Outport
  wires:
  In1/1 -> Switch1/1, Compare To Constant1/1
  Compare To Constant1/1 -> Switch1/2
  zero1/1 -> Switch1/3
  Switch1/1 -> Out1/1

== system controller13_AIS/Adaptive Controller 2/adaptive system/integrator/start ramp ==
  0.8 : Constant  Value=mdl.s_delay
  2 : Constant  Value=mdl.i_delay
  Add1 : Sum
  Add2 : Sum  Inputs=+-
  Compare To Zero : simulink/Logic and Bit Operations/Compare To Zero  relop=>  OutDataTypeStr=uint8  ZeroCross=off
  Data Type Conversion : DataTypeConversion
  constant : Constant
  counter : DiscreteIntegrator  gainval=1  SampleTime=-1  UpperSaturationLimit=1  LowerSaturationLimit=0  ICPrevOutput=DiscIntNeverNeededParam  ICPrevScaledInput=DiscIntNeverNeededParam
  saturation ramp : DiscreteIntegrator  gainval=5  SampleTime=-1  LimitOutput=on  UpperSaturationLimit=1  LowerSaturationLimit=-1  ICPrevOutput=DiscIntNeverNeededParam  ICPrevScaledInput=DiscIntNeverNeededParam
  Out1 : Outport
  wires:
  constant/1 -> counter/1
  2/1 -> Add1/1
  0.8/1 -> Add1/2
  counter/1 -> Add2/1
  Add1/1 -> Add2/2
  Add2/1 -> Compare To Zero/1
  Compare To Zero/1 -> Data Type Conversion/1
  saturation ramp/1 -> Out1/1
  Data Type Conversion/1 -> saturation ramp/1

== system controller13_AIS/Adaptive Controller 2/attitude and thrust controller/Yaw Controller/start ramp ==
  0.8 : Constant  Value=0.01
  2 : Constant  Value=mdl.i_delay
  Add1 : Sum
  Add2 : Sum  Inputs=+-
  Compare To Zero : simulink/Logic and Bit Operations/Compare To Zero  relop=>  OutDataTypeStr=uint8  ZeroCross=off
  Data Type Conversion : DataTypeConversion
  constant : Constant
  counter : DiscreteIntegrator  gainval=1  SampleTime=-1  UpperSaturationLimit=1  LowerSaturationLimit=0  ICPrevOutput=DiscIntNeverNeededParam  ICPrevScaledInput=DiscIntNeverNeededParam
  saturation ramp : DiscreteIntegrator  gainval=5  SampleTime=-1  LimitOutput=on  UpperSaturationLimit=1  LowerSaturationLimit=-1  ICPrevOutput=DiscIntNeverNeededParam  ICPrevScaledInput=DiscIntNeverNeededParam
  Out1 : Outport
  wires:
  constant/1 -> counter/1
  2/1 -> Add1/1
  0.8/1 -> Add1/2
  counter/1 -> Add2/1
  Add1/1 -> Add2/2
  Add2/1 -> Compare To Zero/1
  Compare To Zero/1 -> Data Type Conversion/1
  saturation ramp/1 -> Out1/1
  Data Type Conversion/1 -> saturation ramp/1

== system controller13_AIS/Adaptive Controller 2/observer/Rotaion/filtered derivative ==
  In1 : Inport
  att_s : Gain  Gain=mdl.f1
  filtered derivative : simulink/Discrete/Transfer Fcn Lead or Lag  PoleZ=mdl.zf1  ZeroZ=1  ICPrevOutput=0.0  ICPrevInput=0.0  DoSatur=off
      settings: SourceProductBaseCode=SL
  low pass3 : DiscreteTransferFcn  Numerator=mdl.vlp.n  Denominator=mdl.vlp.d
  Out1 : Outport
  wires:
  filtered derivative/1 -> low pass3/1
  att_s/1 -> filtered derivative/1
  In1/1 -> att_s/1
  low pass3/1 -> Out1/1

== system controller13_AIS/Adaptive Controller 2/observer/lateral observer/saturation ==
  In1 : Inport
  MinMax2 : MinMax  Inputs=2
  MinMax3 : MinMax  Function=max  Inputs=2
  lw1 : Constant  Value=-mdl.fd_lim
  up1 : Constant  Value=mdl.fd_lim
  Out1 : Outport
  wires:
  In1/1 -> MinMax2/2
  up1/1 -> MinMax2/1
  lw1/1 -> MinMax3/1
  MinMax2/1 -> MinMax3/2
  MinMax3/1 -> Out1/1

== system controller13_AIS/Adaptive Controller 2/observer1/UKF/UKF_inner ==
  z_raw : Inport
  f_cmd : Inport  Port=2
  tau_cmd_x : Inport  Port=3
  tau_cmd_y : Inport  Port=4
  Delay : Delay  DelayLength=1  InitialCondition="reshape((   diag(vertcat(   1e-4 * ones(12,1),   [0.107 * 7.2e-4; 0.107 * 7.2e-4; 0.107 * 7.2e-4],   [1.1e-21; 1.1e-21; 1e-21]   ))   )',   1,   []   )'"  SampleTime=mdl.T
  Delay1 : Delay  DelayLength=1  InitialCondition=vertcat( [0;0;0], [1;0;0;0], [0;0;0], [0;0;0], [0.981 * 7.2e-4; 0.981 * 7.2e-4; 0.981 * 7.2e-4], [5e-6;5e-6;0] )  SampleTime=mdl.T
  Delay2 : Delay  DelayLength=1  InitialCondition=zeros(13,1)  SampleTime=mdl.T
  Delay3 : Delay  DelayLength=1  InitialCondition=0  SampleTime=mdl.T
  To Workspace3 : ToWorkspace  VariableName=ukf_P_flats  SaveFormat=Timeseries  SampleTime=-1
  UKF update then predict : MATLAB Function  TreatAsAtomicUnit=on  mask{sys=ukf_sys}
  s_out : Outport
  wires:
  z_raw/1 -> UKF update then predict/1(z_raw), Delay2/1
  f_cmd/1 -> UKF update then predict/3(f_cmd)
  tau_cmd_x/1 -> UKF update then predict/4(tau_cmd_x)
  tau_cmd_y/1 -> UKF update then predict/5(tau_cmd_y)
  UKF update then predict/1(s_out) -> s_out/1, Delay1/1
  UKF update then predict/2(P_out_flat) -> Delay/1
  Delay/1 -> UKF update then predict/7(P_in_flat), To Workspace3/1
  Delay1/1 -> UKF update then predict/6(s_in)
  Delay2/1 -> UKF update then predict/2(z_raw_prev)
  UKF update then predict/3(is_init_out) -> Delay3/1
  Delay3/1 -> UKF update then predict/8(is_init_in)

== system controller13_AIS/Adaptive Controller 2/observer1/UKF1/UKF_inner ==
  z_raw : Inport
  f_cmd : Inport  Port=2
  tau_cmd_x : Inport  Port=3
  tau_cmd_y : Inport  Port=4
  s_prediction_time : Inport  Port=5
  Delay : Delay  DelayLength=1  InitialCondition=ukf_P0_flat  SampleTime=mdl.T
  Delay1 : Delay  DelayLength=1  InitialCondition=ukf_s0  SampleTime=mdl.T
  Delay2 : Delay  DelayLength=1  InitialCondition=[0,0,0, 1,0,0,0,0, 0,0,0, 0,0]'  SampleTime=mdl.T
  Delay3 : Delay  DelayLength=1  InitialCondition=0  SampleTime=mdl.T
  Terminator : Terminator
  To Workspace3 : ToWorkspace  VariableName=ukf_P_flats  SaveFormat=Timeseries  SampleTime=-1
  UKF update then predict : MATLAB Function  TreatAsAtomicUnit=on  mask{sys=ukf_sys}
  bee cov to SI cov : MATLAB Function  TreatAsAtomicUnit=on
  bee units to SI : MATLAB Function  TreatAsAtomicUnit=on
  bee units to SI1 : MATLAB Function  TreatAsAtomicUnit=on
  s_prediction_out : Outport
  s_out : Outport  Port=2
  wires:
  z_raw/1 -> Delay2/1, UKF update then predict/1(z_raw)
  f_cmd/1 -> UKF update then predict/3(f_cmd)
  tau_cmd_x/1 -> UKF update then predict/4(tau_cmd_x)
  tau_cmd_y/1 -> UKF update then predict/5(tau_cmd_y)
  UKF update then predict/1(s_out) -> Delay1/1, bee units to SI/1(s_bee)
  UKF update then predict/2(P_out_flat) -> Delay/1
  Delay/1 -> UKF update then predict/7(P_in_flat), bee cov to SI cov/1(P_flat_bee)
  Delay1/1 -> UKF update then predict/6(s_in)
  Delay2/1 -> UKF update then predict/2(z_raw_prev)
  UKF update then predict/3(is_init_out) -> Delay3/1
  Delay3/1 -> UKF update then predict/8(is_init_in)
  UKF update then predict/4(s_out_pre) -> Terminator/1
  bee units to SI/1(s_si) -> s_out/1  "UKF states"
  bee cov to SI cov/1(P_flat_si) -> To Workspace3/1  "UKF P flats"
  UKF update then predict/5(s_prediction_out) -> bee units to SI1/1(s_bee)
  s_prediction_time/1 -> UKF update then predict/9(s_prediction_time)
  bee units to SI1/1(s_si) -> s_prediction_out/1  "UKF states prediction"

== system controller13_AIS/Adaptive Controller 2/observer1/UKF2/UKF_inner ==
  z_raw : Inport
  f_cmd : Inport  Port=2
  tau_cmd_x : Inport  Port=3
  tau_cmd_y : Inport  Port=4
  Delay : Delay  DelayLength=1  InitialCondition="reshape((   diag(vertcat(   1e-4 * ones(12,1),   [0.107 * 7.2e-4; 0.107 * 7.2e-4; 0.107 * 7.2e-4],   [1.1e-21; 1.1e-21; 1e-21]   ))   )',   1,   []   )'"  SampleTime=mdl.T
  Delay1 : Delay  DelayLength=1  InitialCondition=vertcat( [0;0;0], [1;0;0;0], [0;0;0], [0;0;0], [0.981 * 7.2e-4; 0.981 * 7.2e-4; 0.981 * 7.2e-4], [5e-6;5e-6;0] )  SampleTime=mdl.T
  Delay2 : Delay  DelayLength=1  InitialCondition=zeros(13,1)  SampleTime=mdl.T
  Delay3 : Delay  DelayLength=1  InitialCondition=0  SampleTime=mdl.T
  To Workspace3 : ToWorkspace  VariableName=ukf_P_flats  SaveFormat=Timeseries  SampleTime=-1
  UKF update then predict : MATLAB Function  TreatAsAtomicUnit=on  mask{sys=ukf_sys}
  s_out : Outport
  wires:
  z_raw/1 -> UKF update then predict/1(z_raw), Delay2/1
  f_cmd/1 -> UKF update then predict/3(f_cmd)
  tau_cmd_x/1 -> UKF update then predict/4(tau_cmd_x)
  tau_cmd_y/1 -> UKF update then predict/5(tau_cmd_y)
  UKF update then predict/1(s_out) -> s_out/1, Delay1/1
  UKF update then predict/2(P_out_flat) -> Delay/1
  Delay/1 -> UKF update then predict/7(P_in_flat), To Workspace3/1
  Delay1/1 -> UKF update then predict/6(s_in)
  Delay2/1 -> UKF update then predict/2(z_raw_prev)
  UKF update then predict/3(is_init_out) -> Delay3/1
  Delay3/1 -> UKF update then predict/8(is_init_in)

== system controller13_AIS/Adaptive Controller 2/observer1/lateral observer/saturation ==
  In1 : Inport
  MinMax2 : MinMax  Inputs=2
  MinMax3 : MinMax  Function=max  Inputs=2
  lw1 : Constant  Value=-mdl.fd_lim
  up1 : Constant  Value=mdl.fd_lim
  Out1 : Outport
  wires:
  In1/1 -> MinMax2/2
  up1/1 -> MinMax2/1
  lw1/1 -> MinMax3/1
  MinMax2/1 -> MinMax3/2
  MinMax3/1 -> Out1/1

== matlab function controller13_AIS/Adaptive Controller 1/adaptive setpoint rd ==
  data: rd output; rd_d output; rd_dd output; rd_ddd output; rd_dddd output; time input; r input; r_d input; landing input; som_ph input; ctr1 parameter; som parameter; mdl parameter
function [rd,rd_d,rd_dd,rd_ddd,rd_dddd] = fcn(time, r, r_d, landing,som_ph, ctr1, som, mdl)
%#codegen

rd = [ctr1.setpoint.x; ctr1.setpoint.y; ctr1.setpoint.z];
rd_d = zeros(3,1);
rd_dd = zeros(3,1);
rd_ddd = zeros(3,1);
rd_dddd = zeros(3,1);

if time <= mdl.i_delay+0.1
    rd_z = ctr1.takeoff.height;
    rd   = [ctr1.setpoint.x; ctr1.setpoint.y; rd_z];
end

% takeoff
if ctr1.takeoff.en
    if time > mdl.i_delay+0.1 && time < (mdl.i_delay+0.1+ctr1.takeoff.time)
        rd_z = ctr1.takeoff.height + (((ctr1.setpoint.z-ctr1.takeoff.height)/ctr1.takeoff.time)*(time-mdl.i_delay-0.1));
        if rd_z > ctr1.setpoint.z
            rd_z = ctr1.setpoint.z;
        end
        rd   = [ctr1.setpoint.x; ctr1.setpoint.y; rd_z];
    end
end

% planned landing 
if ctr1.landing.en
    if time > (mdl.rt-ctr1.landing.time)
        rd_z = ctr1.setpoint.z-(((ctr1.setpoint.z-ctr1.landing.height)/ctr1.landing.time)*(time-mdl.rt+ctr1.landing.time));
        if rd_z < ctr1.landing.height
            rd_z = ctr1.landing.height;
        end
        rd   = [ctr1.setpoint.x; ctr1.setpoint.y; rd_z];
    end
end

% forced landing
if landing
    rd_z = 0.02;
    rd   = [ctr1.setpoint.x; ctr1.setpoint.y; rd_z];
end


% somersault
if som.en
    if time > som.t_start + som.t_rise + som.t_acc + som.t_dcc + som.t_rec
        % % afterwards 
        %dt = som.t_start + som.t_rise + som.t_acc + som.t_dcc + som.t_rec - time;
        %rd = rd + dt*(r-rd);
    elseif time > som.t_start + som.t_rise + som.t_acc + som.t_dcc
        % recovery
        dt = som.t_start + som.t_rise + som.t_acc + som.t_dcc + som.t_rec - time;
        rd = rd + (dt/som.t_rec)*(r-rd);
        rd_d = rd_d + 0.5*(dt/som.t_rec)*(r_d-rd_d);
        rd(1) = min(max(rd(1),-0.25),0.25); % 25 cm envelope
        rd(2) = min(max(rd(2),-0.25),0.25); % 25 cm envelope
        rd(3) = max(rd(3),0.02); % min altitude setpoint.
    end
end


end

== matlab function controller13_AIS/Force//Torque to Trajectory Specs 1/nominal desired voltage/force to voltage (hovering) /MATLAB Function ==
  data: Vi input; Vo output; mdl parameter; ctr1 parameter
function Vo = fcn(Vi,mdl,ctr1)
%old script
% if max(Vi)>mdl.max_v
%     Vo = Vi * mdl.max_v/max(Vi);
%     % scale down all votages if one exceeds the max limit.
% else
%     Vo = Vi;
% end

%new change (modify max_v to a vector so each DEA has its own max)
% scale_down_ratio_vec = Vi ./ mdl.max_v_vec;
% scale_down_ratio = max(scale_down_ratio_vec);
% bool_scale_down = scale_down_ratio>1;
% 
% if bool_scale_down
%    Vo = Vi/scale_down_ratio;
% else
%    Vo = Vi; 
% end

min_v_vec = mdl.hovering_vec -150;
scale_down_ratio_vec = (Vi-min_v_vec)./(ctr1.safety.volt-min_v_vec);

scale_down_ratio = max(scale_down_ratio_vec);
bool_scale_down = scale_down_ratio>1;

if bool_scale_down
    Vo = min_v_vec + (Vi - min_v_vec)./scale_down_ratio;	
else
	  Vo = Vi; 
end


%extra layer of safety
for i=1:length(Vo)
	Vo(i) = min(Vo(i),ctr1.safety.volt(i));
end
